simulink model "adaptive_mrac_comp"  (R2020a)
settings: Solver=FixedStepAuto  StartTime=0.0  StopTime=89.99  FixedStep=0.01  RelTol=1e-3
values from neighbouring files (symbols this model uses):
  gamma_r = 0.03    [cases_test.m]    (also in cases_tests_lr.m = gamma_r_0 * i; mrac_model_const_ref.m = params(6); mrac_model_lr.m = params(5); mrac_model_lr_init.m = params(8))
  gamma_x = [0.5; 0.5]    [cases_test.m]    (also in cases_tests_lr.m = gamma_x_0 * i; mrac_model_const_ref.m = params(4:5); mrac_model_e2y.m = params(7:8); mrac_model_e2y_2delay.m = params(7:8))
  k_x0 = k_x0_list(:, plant_case)    [cases_test.m]    (also in mrac_model_const_ref.m = [-params(1); params(2)]; mrac_model_e2y.m = params(1:2); mrac_model_e2y_2delay.m = params(1:2); mrac_model_lr_init.m = [-params(1); params(2)])
  P = lyap(ref_sys.A', eye(2))    [cases_test.m]    (also in cases_tests_lr.m; mrac_model_e2y.m = [10, .2; 10, .2]; mrac_model_e2y_2delay.m = [1.5, 0; 1.5, 3.5]; mrac_model_lr_init_low_pass_comp.m = params(3:4))
  ref_sys = canon(ref_sys, 'modal')    [cases_test.m]    (also in cases_tests_lr.m; mrac_model.m = ss([tf_cl_pade; s*tf_cl_pade]); mrac_model_e2y.m = ss([tf_cl_pade; s*tf_cl_pade]); mrac_model_e2y_2delay.m = ss([tf_cl_pade; s*tf_cl_pade]))
undefined symbols (not defined in the file or in its folder): case_, K_r0, ref_x0
settings Model: OrderedModelArguments=off  Creator=lorenzoterenzi  LastModifiedBy=lorenzoterenzi

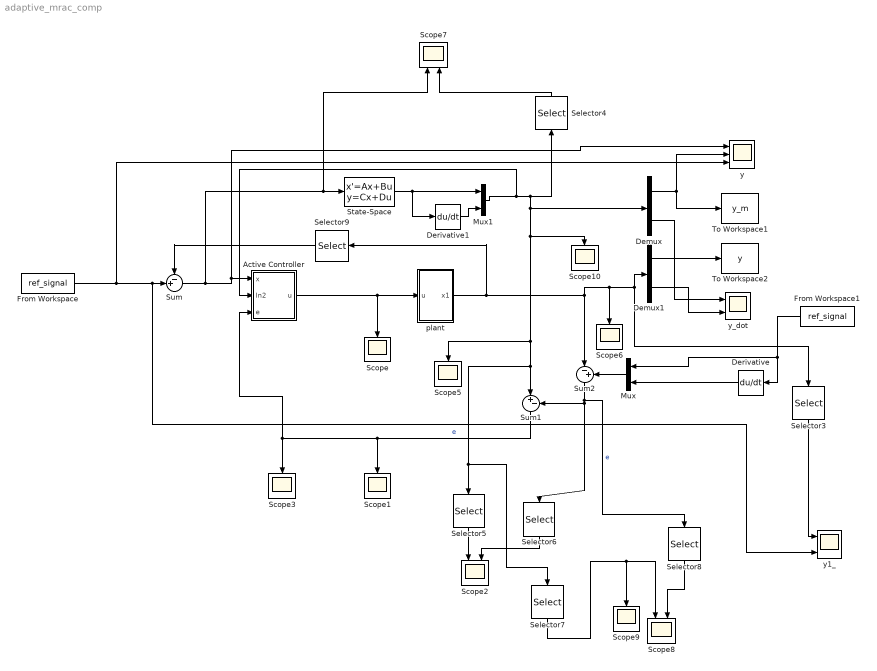
== system adaptive_mrac_comp ==
  Active Controller : Subsystem
  Demux : Demux  Outputs=2
  Demux1 : Demux  Outputs=2
  Derivative : Derivative
  Derivative1 : Derivative
  From Workspace : FromWorkspace  VariableName=ref_signal
  From Workspace1 : FromWorkspace  VariableName=ref_signal
  Mux : Mux  Inputs=2
  Mux1 : Mux  Inputs=2
  Scope{,1,3,5..6,9..10} (7 alike) : Scope
  Scope2 : Scope  NumInputPorts=2
  Scope7 : Scope  NumInputPorts=2
  Scope8 : Scope  NumInputPorts=2
  Selector{3..6,9} (5 alike) : Selector  InputPortWidth=2  IndexOptions=Index vector (dialog)  Indices=[1]  OutputSizes=1
  Selector7 : Selector  InputPortWidth=2  IndexOptions=Index vector (dialog)  Indices=[2]  OutputSizes=1
  Selector8 : Selector  InputPortWidth=2  IndexOptions=Index vector (dialog)  Indices=[2]  OutputSizes=1
  State-Space : StateSpace  A=ref_sys.A  B=ref_sys.B  C=ref_sys.C  D=ref_sys.D  InitialCondition=ref_x0
  Sum : Sum  Inputs=-+|
  Sum1 : Sum  Inputs=|+-
  Sum2 : Sum  Inputs=|-+
  To Workspace1 : ToWorkspace  VariableName=y_m  SaveFormat=Timeseries  SampleTime=-1
  To Workspace2 : ToWorkspace  VariableName=y  SaveFormat=Timeseries  SampleTime=-1
  plant : Subsystem
  y : Scope  NumInputPorts=3
  y1_ : Scope  NumInputPorts=3
  y_dot : Scope  NumInputPorts=2
  wires:
  Demux/2 -> y_dot/1
  Sum1/1 -> Active Controller/3(e), Scope3/1, Scope1/1  "e"
  Demux1/2 -> y_dot/2
  Demux/1 -> y/2, To Workspace1/1
  Demux1/1 -> To Workspace2/1
  Sum/1 -> State-Space/1, Scope7/1, y/1, Active Controller/1(x)
  Active Controller/1(u) -> plant/1(u), Scope/1
  Selector3/1 -> y1_/1
  From Workspace/1 -> y/3, y1_/3, Sum/2
  plant/1(x1) -> Selector9/1, Scope6/1, Demux1/1, Selector3/1, Sum2/1
  From Workspace1/1 -> Derivative/1, Mux/1
  Mux/1 -> Sum2/2
  Selector4/1 -> Scope7/2
  Selector5/1 -> Scope2/1
  Selector6/1 -> Scope2/2
  Mux1/1 -> Active Controller/2(In2), Scope10/1, Scope5/1, Selector7/1, Selector5/1, Sum1/1, Demux/1, Selector4/1
  Derivative/1 -> Mux/2
  Sum2/1 -> Sum1/2, Selector6/1, Selector8/1  "e"
  Selector7/1 -> Scope9/1, Scope8/1
  Selector8/1 -> Scope8/2
  State-Space/1 -> Derivative1/1, Mux1/1
  Derivative1/1 -> Mux1/2
  Selector9/1 -> Sum/1

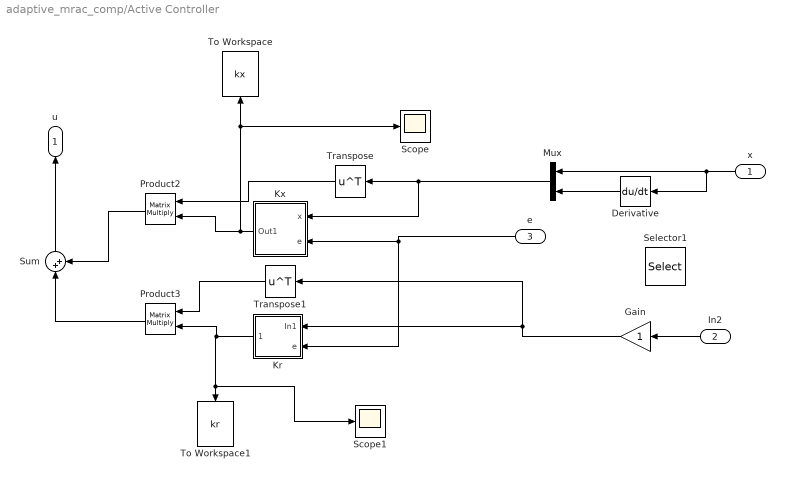
== system adaptive_mrac_comp/Active Controller ==
  x : Inport
  In2 : Inport  Port=2
  e : Inport  Port=3
  Derivative : Derivative
  Gain : Gain
  Kr : Subsystem
  Kx : Subsystem
  Mux : Mux  Inputs=2
  Product2 : Product  Multiplication=Matrix(*)
  Product3 : Product  Multiplication=Matrix(*)
  Scope : Scope
  Scope1 : Scope
  Selector1 : Selector  InputPortWidth=2  IndexOptions=Index vector (dialog)  Indices=[1]  OutputSizes=1
  Sum : Sum  Inputs=|++
  To Workspace : ToWorkspace  VariableName=kx  SaveFormat=Timeseries  SampleTime=-1
  To Workspace1 : ToWorkspace  VariableName=kr  SaveFormat=Timeseries  SampleTime=-1
  Transpose : Math  Operator=transpose  SaturateOnIntegerOverflow=on
  Transpose1 : Math  Operator=transpose  SaturateOnIntegerOverflow=on
  u : Outport
  wires:
  Kx/1(Out1) -> Product2/2, To Workspace/1, Scope/1
  Product2/1 -> Sum/2
  Product3/1 -> Sum/1
  e/1 -> Kx/2(e), Kr/2(e)
  Sum/1 -> u/1
  Kr/1(Out1) -> Product3/2, Scope1/1, To Workspace1/1
  In2/1 -> Gain/1
  x/1 -> Derivative/1, Mux/1
  Derivative/1 -> Mux/2
  Mux/1 -> Transpose/1, Kx/1(x)
  Transpose/1 -> Product2/1
  Transpose1/1 -> Product3/1
  Gain/1 -> Kr/1(In1), Transpose1/1

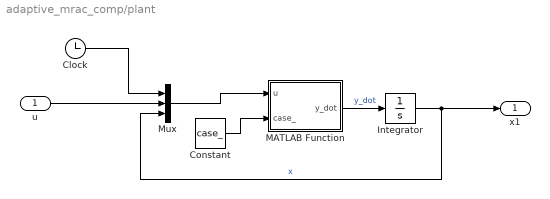
== system adaptive_mrac_comp/plant ==
  u : Inport
  Clock : Clock
  Constant : Constant  Value=case_
  Integrator : Integrator  InitialCondition=[0;0]
  MATLAB Function : MATLAB Function  TreatAsAtomicUnit=on
  Mux : Mux  Inputs=3
  x1 : Outport
  wires:
  Mux/1 -> MATLAB Function/1(u)
  Integrator/1 -> x1/1, Mux/3  "x"
  MATLAB Function/1(y_dot) -> Integrator/1  "y_dot"
  Clock/1 -> Mux/1
  Constant/1 -> MATLAB Function/2(case_)
  u/1 -> Mux/2

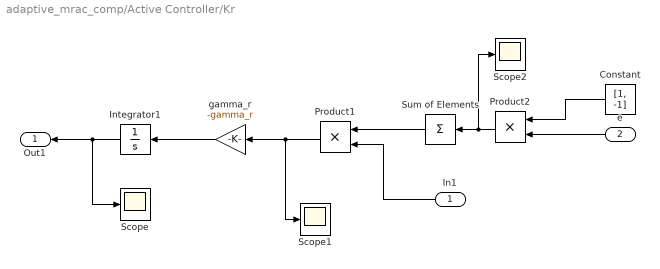
== system adaptive_mrac_comp/Active Controller/Kr ==
  In1 : Inport
  e : Inport  Port=2
  Constant : Constant  Value=[1, -1]
  Integrator1 : Integrator  InitialCondition=K_r0
  Product1 : Product
  Product2 : Product
  Scope : Scope
  Scope1 : Scope
  Scope2 : Scope
  Sum of Elements : Sum  Inputs=+
  gamma_r : Gain  Gain=-gamma_r
  Out1 : Outport
  wires:
  In1/1 -> Product1/2
  Product1/1 -> Scope1/1, gamma_r/1
  Product2/1 -> Scope2/1, Sum of Elements/1
  e/1 -> Product2/2
  Sum of Elements/1 -> Product1/1
  Integrator1/1 -> Out1/1, Scope/1
  Constant/1 -> Product2/1
  gamma_r/1 -> Integrator1/1

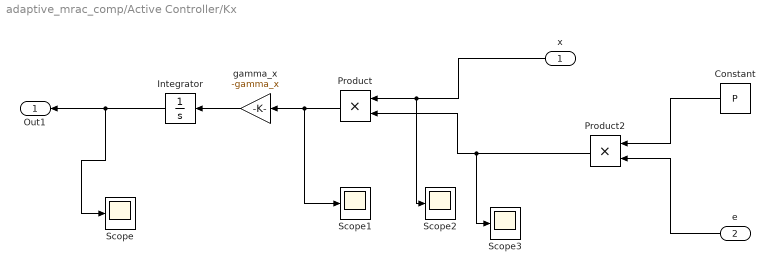
== system adaptive_mrac_comp/Active Controller/Kx ==
  x : Inport
  e : Inport  Port=2
  Constant : Constant  Value=P
  Integrator : Integrator  InitialCondition=k_x0
  Product : Product
  Product2 : Product
  Scope{,1..3} (4 alike) : Scope
  gamma_x : Gain  Gain=-gamma_x
  Out1 : Outport  PortDimensions=[2, 1]
  wires:
  x/1 -> Scope2/1, Product/1
  e/1 -> Product2/2
  Product2/1 -> Scope3/1, Product/2
  Integrator/1 -> Scope/1, Out1/1
  Constant/1 -> Product2/1
  gamma_x/1 -> Integrator/1
  Product/1 -> Scope1/1, gamma_x/1

== matlab function adaptive_mrac_comp/plant/MATLAB Function ==
  data: u input size=4; y_dot output size=2; case_ input
function y_dot = fcn(u, case_)
    t = u(1);
    u_c = u(2);
    y_prev = u(3:4);
    y_dot = models.peter_plant(case_, t, u_c, y_prev);
end


% function y_dot = peter_plant(case_, t, u, y_prev)
%     % case 1: first to second order system transition
%     if case_ == 1
%         M = -1;
%         G = -100;
%     % case 2: second to first order transition
%     elseif case_ == 2 
%         M = 91;
%         G = 100;
%     elseif case_ == 3    
%         M = 50;
%         G = 0.5;
%     elseif case_ == 4
%         M = 50;
%         G = 100;
%     else
%         G = 0;
%         M = 0;
%     end
% 
%     omega_b1 = 6;
%     omega_b2 = 0.2;
%     k_c1 = 90;
%     k_c2 = 30;
% 
%     omega_b = omega_b1 + (omega_b2 - omega_b1)./(1 + exp(-G * (t - M)));
%     k_c = k_c1 + (k_c2 - k_c1)./(1 + exp(-G * (t - M)));
% 
%     A = [0, 1; 0, omega_b];
%     B = [0; k_c];
%     y_dot = A*y_prev + B*u;
% end
